simulink subsystem "s0311_alpha_controller_PP"  (R2019b)
settings: Solver=VariableStepAuto  StartTime=0.0  StopTime=10.0  RelTol=1e-3
model mask{p1=0, p2=0}
  mask prompts: p1 "Position 1st pole"; p2 "Position 2nd pole"
undefined symbols (not defined in the file): PARAMS
libraries: simulink x1
settings Model: Creator=francescoceresetti  LastModifiedBy=paolo

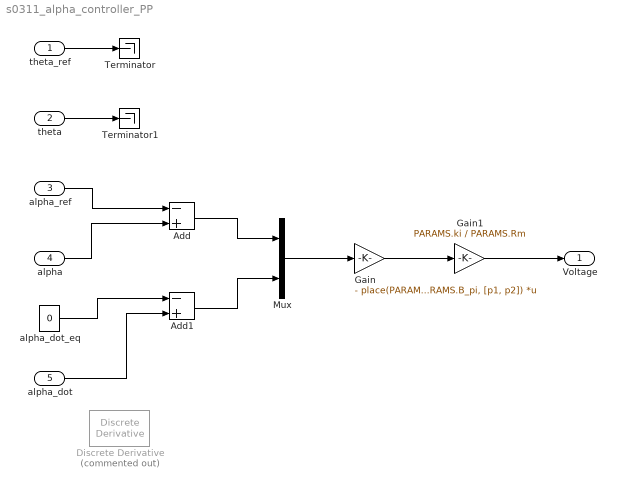
== system s0311_alpha_controller_PP ==
  theta_ref : Inport
  theta : Inport  Port=2
  alpha_ref : Inport  Port=3
  alpha : Inport  Port=4
  "alpha_dot " : Inport  Port=5
  Add : Sum  Inputs=-+
  Add1 : Sum  Inputs=-+
  Discrete Derivative : simulink/Discrete/Discrete Derivative  Commented=on  gainval=1.0  ICPrevScaledInput=0.0  OutMin=[]  OutMax=[]  OutDataType=fixdt(1, 16)  OutScaling=2^-10  DoSatur=off
  Gain : Gain  Gain=- place(PARAMS.A_pi, PARAMS.B_pi, [p1, p2])  Multiplication=Matrix(K*u)
  Gain1 : Gain  Gain=PARAMS.ki / PARAMS.Rm
  Mux : Mux  Inputs=2
  Terminator : Terminator
  Terminator1 : Terminator
  "alpha_dot_eq " : Constant  Value=0
  Voltage : Outport
  wires:
  theta_ref/1 -> Terminator/1
  theta/1 -> Terminator1/1
  alpha_ref/1 -> Add/1
  alpha/1 -> Add/2
  Mux/1 -> Gain/1
  Add/1 -> Mux/1
  Gain/1 -> Gain1/1
  Gain1/1 -> Voltage/1
  "alpha_dot_eq "/1 -> Add1/1
  "alpha_dot "/1 -> Add1/2
  Add1/1 -> Mux/2
